simulink model "JointPosControl5bar"  (R2018b)
settings: Solver=VariableStepAuto  StartTime=0.0  StopTime=10  RelTol=1e-3
libraries: simulink x2
settings Model: Creator=Srikar  LastModifiedBy=holyCow
settings SFSimCC: SimUseLocalCustomCode=off
settings RTWCC: RTWUseLocalCustomCode=off

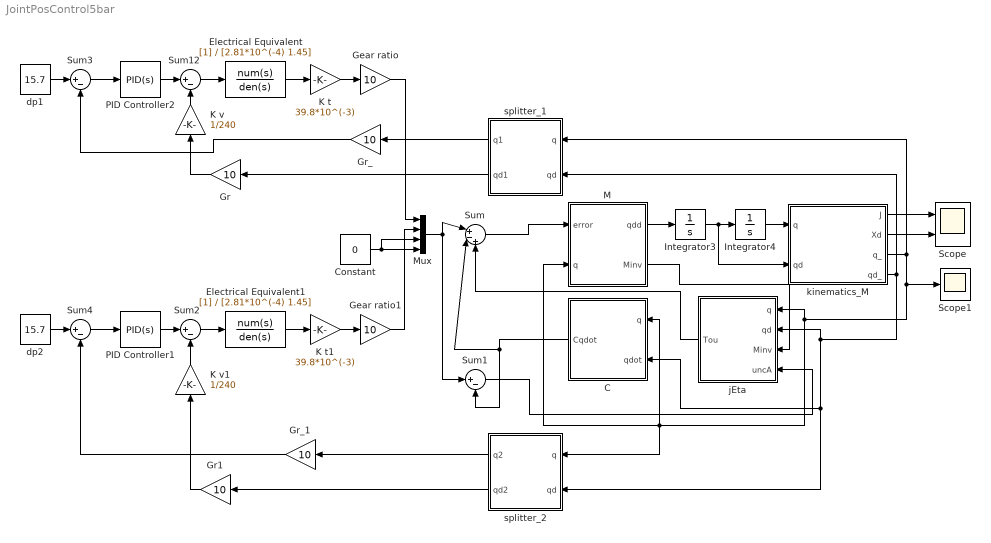
== system JointPosControl5bar ==
  C : MATLAB Function  TreatAsAtomicUnit=on
  Constant : Constant  Value=0
  Electrical Equivalent : TransferFcn  Denominator=[2.81*10^(-4) 1.45]
  Electrical Equivalent1 : TransferFcn  Denominator=[2.81*10^(-4) 1.45]
  Gear ratio : Gain  Gain=10
  Gear ratio1 : Gain  Gain=10
  Gr : Gain  Gain=10
  Gr1 : Gain  Gain=10
  Gr_ : Gain  Gain=10
  Gr_1 : Gain  Gain=10
  Integrator3 : Integrator  InitialCondition=[0 0 0 0]'
  Integrator4 : Integrator  InitialCondition=[0 0 0 0]'
  K t : Gain  Gain=39.8*10^(-3)
  K t1 : Gain  Gain=39.8*10^(-3)
  K v : Gain  Gain=1/240
  K v1 : Gain  Gain=1/240
  M : MATLAB Function  TreatAsAtomicUnit=on
  Mux : Mux
  PID Controller1 : simulink/Continuous/PID Controller  Controller=PID  Form=Parallel  TimeDomain=Continuous-time  SampleTime=-1  IntegratorMethod=Forward Euler  FilterMethod=Forward Euler  ControllerParametersSource=internal  P=4.03915691539375  I=47.1446499264724  D=0.0745984943668176  UseFilter=on  N=1888.25178733024  TunerSelectOption=Transfer Function Based (PID Tuner App)  InitialConditionSource=internal  InitialConditionForIntegrator=0  InitialConditionForFilter=0  DifferentiatorICPrevScaledInput=0  ExternalReset=none  TrackingMode=off  Kt=1  LimitOutput=off  UpperSaturationLimit=inf  LowerSaturationLimit=-inf  LinearizeAsGain=on  AntiWindupMode=none  Kb=1  POutMin=[]  POutMax=[]  IOutMin=[]  IOutMax=[]  DOutMin=[]  DOutMax=[]  NOutMin=[]  NOutMax=[]  SumOutMin=[]  SumOutMax=[]  SaturationOutMin=[]  SaturationOutMax=[]  PParamMin=[]  PParamMax=[]  IParamMin=[]  IParamMax=[]  DParamMin=[]  DParamMax=[]  NParamMin=[]  NParamMax=[]  KbParamMin=[]  KbParamMax=[]  KtParamMin=[]  KtParamMax=[]  KbOutMin=[]  KbOutMax=[]  KtOutMin=[]  KtOutMax=[]  IntegratorOutMin=[]  IntegratorOutMax=[]  FilterOutMin=[]  FilterOutMax=[]  SumI1OutMin=[]  SumI1OutMax=[]  SumI2OutMin=[]  SumI2OutMax=[]  SumI3OutMin=[]  SumI3OutMax=[]  SumI4OutMin=[]  SumI4OutMax=[]  SumDOutMin=[]  SumDOutMax=[]  DifferentiatorOutMin=[]  DifferentiatorOutMax=[]  FilterDiffOutCoefMin=[]  FilterDiffOutCoefMax=[]  ReciprocalOutMin=[]  ReciprocalOutMax=[]  SumDenOutMin=[]  SumDenOutMax=[]  SumNumOutMin=[]  SumNumOutMax=[]  DivideOutMin=[]  DivideOutMax=[]  IntegratorContinuousStateAttributes=''  IntegratorStateMustResolveToSignalObject=off  IntegratorRTWStateStorageClass=Auto  FilterContinuousStateAttributes=''  FilterStateMustResolveToSignalObject=off  FilterRTWStateStorageClass=Auto  ParallelPVariant=InternalParameters  IdealPVariant=Disabled  IVariant=InternalParameters  DVariant=InternalParameters  IntegratorVariant=Continuous  SatVariant=Disabled  AWVariant=Passthrough  PCopyVariant=Disabled  TRVariant=Disabled  FdbkBlocksVariant=Forward  IdealPFdbkVariant=Disabled  SatFdbkVariant=Disabled  DerivativeFilterVariant=ContFilter  NVariant=InternalParameters  NCopyVariant=Disabled  FilterICVariant=InternalICsFilter  IntegratorICVariant=InternalICs  ExternalResetVariant=Disabled  TRSumVariant=Passthrough  SumFdbkVariant=Disabled  SumVariant=Sum_PID
  PID Controller2 : simulink/Continuous/PID Controller  Controller=PID  Form=Parallel  TimeDomain=Continuous-time  SampleTime=-1  IntegratorMethod=Forward Euler  FilterMethod=Forward Euler  ControllerParametersSource=internal  P=4.03915691539375  I=47.1446499264724  D=0.0745984943668176  UseFilter=on  N=1888.25178733024  TunerSelectOption=Transfer Function Based (PID Tuner App)  InitialConditionSource=internal  InitialConditionForIntegrator=0  InitialConditionForFilter=0  DifferentiatorICPrevScaledInput=0  ExternalReset=none  TrackingMode=off  Kt=1  LimitOutput=off  UpperSaturationLimit=inf  LowerSaturationLimit=-inf  LinearizeAsGain=on  AntiWindupMode=none  Kb=1  POutMin=[]  POutMax=[]  IOutMin=[]  IOutMax=[]  DOutMin=[]  DOutMax=[]  NOutMin=[]  NOutMax=[]  SumOutMin=[]  SumOutMax=[]  SaturationOutMin=[]  SaturationOutMax=[]  PParamMin=[]  PParamMax=[]  IParamMin=[]  IParamMax=[]  DParamMin=[]  DParamMax=[]  NParamMin=[]  NParamMax=[]  KbParamMin=[]  KbParamMax=[]  KtParamMin=[]  KtParamMax=[]  KbOutMin=[]  KbOutMax=[]  KtOutMin=[]  KtOutMax=[]  IntegratorOutMin=[]  IntegratorOutMax=[]  FilterOutMin=[]  FilterOutMax=[]  SumI1OutMin=[]  SumI1OutMax=[]  SumI2OutMin=[]  SumI2OutMax=[]  SumI3OutMin=[]  SumI3OutMax=[]  SumI4OutMin=[]  SumI4OutMax=[]  SumDOutMin=[]  SumDOutMax=[]  DifferentiatorOutMin=[]  DifferentiatorOutMax=[]  FilterDiffOutCoefMin=[]  FilterDiffOutCoefMax=[]  ReciprocalOutMin=[]  ReciprocalOutMax=[]  SumDenOutMin=[]  SumDenOutMax=[]  SumNumOutMin=[]  SumNumOutMax=[]  DivideOutMin=[]  DivideOutMax=[]  IntegratorContinuousStateAttributes=''  IntegratorStateMustResolveToSignalObject=off  IntegratorRTWStateStorageClass=Auto  FilterContinuousStateAttributes=''  FilterStateMustResolveToSignalObject=off  FilterRTWStateStorageClass=Auto  ParallelPVariant=InternalParameters  IdealPVariant=Disabled  IVariant=InternalParameters  DVariant=InternalParameters  IntegratorVariant=Continuous  SatVariant=Disabled  AWVariant=Passthrough  PCopyVariant=Disabled  TRVariant=Disabled  FdbkBlocksVariant=Forward  IdealPFdbkVariant=Disabled  SatFdbkVariant=Disabled  DerivativeFilterVariant=ContFilter  NVariant=InternalParameters  NCopyVariant=Disabled  FilterICVariant=InternalICsFilter  IntegratorICVariant=InternalICs  ExternalResetVariant=Disabled  TRSumVariant=Passthrough  SumFdbkVariant=Disabled  SumVariant=Sum_PID
  Scope : Scope  NumInputPorts=2
  Scope1 : Scope
  Sum : Sum  Inputs=|+-+
  Sum{1..4,12} (5 alike) : Sum  Inputs=|+-
  dp1 : Constant  Value=15.7
  dp2 : Constant  Value=15.7
  jEta : MATLAB Function  TreatAsAtomicUnit=on
  kinematics_M : MATLAB Function  TreatAsAtomicUnit=on
  splitter_1 : MATLAB Function  TreatAsAtomicUnit=on
  splitter_2 : MATLAB Function  TreatAsAtomicUnit=on
  wires:
  Constant/1 -> Mux/3, Mux/4
  Gr/1 -> K v/1
  Electrical Equivalent/1 -> K t/1
  PID Controller2/1 -> Sum12/1
  dp1/1 -> Sum3/1
  Gr_/1 -> Sum3/2
  K v/1 -> Sum12/2
  Sum12/1 -> Electrical Equivalent/1
  K t/1 -> Gear ratio/1
  Sum3/1 -> PID Controller2/1
  Gear ratio/1 -> Mux/1
  splitter_1/1(q1) -> Gr_/1
  splitter_1/2(qd1) -> Gr/1
  Gr_1/1 -> Sum4/2
  K t1/1 -> Gear ratio1/1
  Electrical Equivalent1/1 -> K t1/1
  Sum2/1 -> Electrical Equivalent1/1
  Gr1/1 -> K v1/1
  dp2/1 -> Sum4/1
  K v1/1 -> Sum2/2
  PID Controller1/1 -> Sum2/1
  Sum4/1 -> PID Controller1/1
  Gear ratio1/1 -> Mux/2
  splitter_2/1(q2) -> Gr_1/1
  splitter_2/2(qd2) -> Gr1/1
  kinematics_M/2(Xd) -> Scope/2
  kinematics_M/4(qd_) -> splitter_2/2(qd), C/2(qdot), jEta/2(qd), splitter_1/2(qd)
  Integrator4/1 -> kinematics_M/1(q)
  kinematics_M/1(J) -> Scope/1
  kinematics_M/3(q_) -> splitter_2/1(q), C/1(q), M/2(q), jEta/1(q), Scope1/1, splitter_1/1(q)
  M/1(qdd) -> Integrator3/1
  Sum/1 -> M/1(error)
  Sum1/1 -> jEta/4(uncA)
  C/1(Cqdot) -> Sum/2, Sum1/2
  M/2(Minv) -> jEta/3(Minv)
  jEta/1(Tou) -> Sum/3
  Mux/1 -> Sum/1, Sum1/1
  Integrator3/1 -> kinematics_M/2(qd), Integrator4/1

== matlab function JointPosControl5bar/splitter_1 ==
  data: q input; q1 output; qd input; qd1 output
function [q1, qd1] = fcn(q, qd)
q1 = q(1);
qd1 = qd(1);

== matlab function JointPosControl5bar/C ==
  data: q input; Cqdot output; qdot input
function Cqdot  = fcn(q, qdot)
q1 = q(1);
q2 = q(2);
q3 = q(3);
q4 = q(4);

C=[0.E-307,(-0.234804E-3).*cos(q1).*sin(q2),0.496696E-3.*sin(q1+(-1).*q3),cos(q1).*((-0.234804E-3).*sin(q1)+(-0.234804E-3).*sin(q2));0.234804E-3.*cos(q1).*sin(q2),0.E-307,0,0.234804E-3.*cos(q1).*sin(q2)+(-0.469609E-3).*cos(q2).*sin(q4);(-0.496696E-3).*sin(q1+(-1).*q3),0,0.E-307,0;cos(q1).*(0.234804E-3.*sin(q1)+0.234804E-3.*sin(q2)),0.469609E-3.*cos(q2).*sin(q1)+(0.234804E-3.*cos(q1)+(-0.469609E-3).*cos(q4)).*sin(q2),0,0.234804E-3.*cos(q1).*sin(q1)+(-0.234804E-3).*cos(q4).*sin(q4)];
Cqdot = C*qdot;

== matlab function JointPosControl5bar/splitter_2 ==
  data: q input; q2 output; qd input; qd2 output
function [q2, qd2] = fcn(q, qd)
q2 = q(2);
qd2 = qd(2);

== matlab function JointPosControl5bar/jEta ==
  data: Tou output; q input; qd input; Minv input; uncA input
function Tou  = fcn(q, qd, Minv, uncA)
l = 0.18;
q1 = q(1);
q2 = q(2);
q3 = q(3);
q4 = q(4);

JEta = l .* [sin(q1) -sin(q2) sin(q3) -sin(q4);
                -cos(q1) cos(q2) -cos(q3) cos(q4)];
   
Jdot = l .* [cos(q1) -cos(q2) cos(q3) -cos(q4)
                sin(q1) -sin(q2) sin(q3) -sin(q4)];

B = (JEta * Minv * uncA) + (Jdot * qd);
A = inv(JEta * Minv * JEta');
lambda = -1 * (A * B);

Tou = JEta' * lambda;

== matlab function JointPosControl5bar/M ==
  data: error input; qdd output; q input; Minv output
function [qdd, Minv]  = fcn(error, q)
l=0.18;
q1 = q(1);
q2 = q(2);
q3 = q(3);
q4 = q(4);

m1=0.03285303;
m2=0.02898819;
m3=0.03066024;
m4=0.02898819;
I1=2.19e-006;
I2=1.99e-006;
I3=1.2e-006;
I4=1.99e-006;
Jv1=[(-l/2)*sin(q1) 0 0 0; (l/2)*cos(q1) 0 0 0];
Jv2=[0 (-l/2)*sin(q2) 0 0; 0 (l/2)*cos(q2) 0 0];
Jv3=[-l*sin(q1) 0 (-l/2)*sin(q3) 0; l*cos(q1) 0 (l/2)*cos(q3) 0];
Jv4=[0 -l*sin(q2) 0 (-l/2)*sin(q4); 0 l*cos(q2) 0 (l/2)*cos(q4)];
Jw1=[0 0 0 0;0 0 0 0;1 0 0 0];
Jw2=[0 0 0 0;0 0 0 0;0 1 0 0];
Jw3=[0 0 0 0;0 0 0 0;0 0 1 0];
Jw4=[0 0 0 0;0 0 0 0;0 0 0 1];
M=(Jv1')*m1*(Jv1)+(Jv2')*m2*(Jv2)+(Jv3')*m3*(Jv3)+(Jv4')*m4*(Jv4)+(Jw1')*I1*(Jw1)+(Jw2')*I2*(Jw2)+(Jw3')*I3*(Jw3)+(Jw4')*I4*(Jw4);
% M = (Jw1')*I1*(Jw1)+(Jw2')*I2*(Jw2)+(Jw3')*I3*(Jw3)+(Jw4')*I4*(Jw4);
% M = [1 0 0 0; 0 1 0 0; 0 0 1 0; 0 0 0 1];
Minv=inv(M);
qdd = Minv * error;

== matlab function JointPosControl5bar/kinematics_M ==
  data: q input; J output; Xd output; q_ output; qd_ output; qd input
function [J, Xd, q_, qd_]  = fcn(q, qd)

q1 = q(1);
q2 = q(2);

l = 0.18;
xFlag = 0;
yFlag = 0;

if q1 <= 0
    q1 = 0.1*pi;
end

if q2 <= 0
    q2 = 0.1*pi;
end

if q2 < q1
    q2 = q1;
end

xb = l*cos(q2);
yb = l*sin(q2);
xd = l + l*cos(q1);
yd = l*sin(q1);

dsquare = (xb - xd)^2 + (yb - yd)^2;

%avoiding singularity,
if dsquare >= (2*l)^2
    
    dsquare = (2*l)^2;
    x = sqrt(2*(l^2) + 2*(l^2)*cos(q1));
    alpha = asin((l*sin(q1))/x);
    beta = acos(((x^2) - (3*(l^2)))/(2*l*x));
    
    %we are assuming that q2 is being driven by q1, which can also be the
    %other way around.
    q2 = alpha + beta;
    
    xb = l*cos(q2);
    yb = l*sin(q2);
    
    slope = (sin(q1) - sin(q2))/(1 + cos(q1) - cos(q2));
    q4 = atan2(slope, 1);
    q3 = pi + q4;
    
    %for x and y,
    x = xb + l*cos(q4);
    y = yb + l*sin(q4); % its actually yb - l*sin(q4) but since q4 is already denoted as negative, + is used.
    
    dq4_1 = -cot(q1)/((sec(q4))^2);
    dq4_2 = -cot(q2)/((sec(q4))^2);
    
    dx_1 = -l*sin(q4)*dq4_1;
    dx_2 = -l*sin(q2) -l*sin(q4)*dq4_2;
    
    dy_1 = l*cos(q4)*dq4_1;
    dy_2 = l*cos(q2) + l*cos(q4)*dq4_2;
    
    q4d = (cos(q1)*qd(1) - cos(q2)*qd(2))/(2*cos(q4));
    q3d = q4d;
    
else

    %by Heron's formula
    k = 0.25 * sqrt(((2*l)^2 - dsquare) * (dsquare));
    m = sqrt((2*l)^2 - dsquare);
    
    %considering only the y-coordinate that is above the line joining the
    %centers of the corresponding two circles.
    x = (0.5 * (xb + xd)) + (2 * (yb - yd) * (k/dsquare));
    y = (0.5 * (yb + yd)) + (2 * (xd - xb) * (k/dsquare));
    
    %establishing constraints:
    %for x,
    if x >= 2*l + l*cos(q1)
        x = 2*l + l*cos(q1);
        xFlag = 1;
    elseif x <= l*cos(q1)
        x = l*cos(q1);
        xFlag = 1;
    end
    
    %for y,
    if y >= l + l*sin(q2)
        y = l + l*sin(q2);
        yFlag = 1;
    
    elseif y <= l*sin(q2) - l
        y = l*sin(q2) -l;
        yFlag = 1;
    end
    
    %now for computing q3 and q4,
    q4 = asin((y - (l*sin(q2)))/l);
    q3 = acos((x - l - l*cos(q1))/l);
    
    d = sqrt(dsquare);

    ddq_1 = ((l^2)/d)*(sin(q1 - q2) - sin(q1));
    ddq_2 = ((l^2)/d)*(sin(q2) - sin(q1 - q2));
    
    dL_1 = 2*(l^2)*(sin(q1) - sin(q1 - q2));
    dL_2 = 2*(l^2)*(sin(q1 - q2) - sin(q2));
    
    dK_1 = ((d/(2*m))*dL_1 - m*ddq_1) / (4*dsquare);
    dK_2 = ((d/(2*m))*dL_2 - m*ddq_2) / (4*dsquare);
    
    if xFlag == 0
        dx_1 = -0.5*l*sin(q1) - 2* (k/dsquare) *l*cos(q1) + 2*l*(sin(q2) - sin(q1))*dK_1;
        dx_2 = -0.5*l*sin(q2) + 2* (k/dsquare) *l*cos(q2) + 2*l*(sin(q2) - sin(q1))*dK_2;
    else
        dx_1 = -l*sin(q1);
        dx_2 = 0;
    end
    
    if yFlag == 0
        dy_1 = 0.5*l*cos(q1) - 2* (k/dsquare) *l*sin(q1) + 2*l*(1 + cos(q1) - cos(q2))*dK_1;
        dy_2 = 0.5*l*cos(q2) + 2* (k/dsquare) *l*sin(q2) + 2*l*(1 + cos(q1) - cos(q2))*dK_2;
    else
        dy_1 = 0;
        dy_2 = l*cos(q2);    
    end  
    
    %for q3d and q4d,
    a = sin(q2)*qd(2) - sin(q1)*qd(1);
    b = cos(q1)*qd(1) - cos(q2)*qd(2);
    c = sin(q3)*cos(q4) - sin(q4)*cos(q3);

    q3d = (cos(q4)*a + sin(q4)*b)/c;
    q4d = (sin(q3)*q3d + sin(q1)*qd(1) - sin(q2)*qd(2))/sin(q4);

end

%q5 =  4*pi - (q1 + q2 + q3 + q4);
q_ = [q1; q2; q3; q4];
qd_ = [qd(1); qd(2); q3d; q4d];

Xd = [x; y];

J = [dx_1 dx_2;
     dy_1 dy_2];
